simulink model "Single_Phase_Controlled_FWR_RLslx"  (R2025a)
settings: Solver=ode23tb  StartTime=0.0  StopTime=0.1  MaxStep=1e-4  RelTol=1e-3
libraries: spsThyristorLib x4, spsVoltageMeasurementLib x2, spsACVoltageSourceLib x1, spsCurrentMeasurementLib x1, spsDiodeLib x1, spsMeanLib x1, spsSeriesRLCBranchLib x1, sps_lib x1
settings Model: Creator=Jawad  LastModifiedBy=Jawad

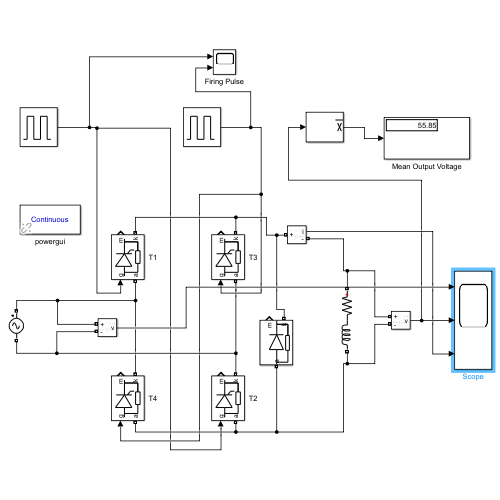
[thumbnail: Simulink's stored preview of the top-level diagram]
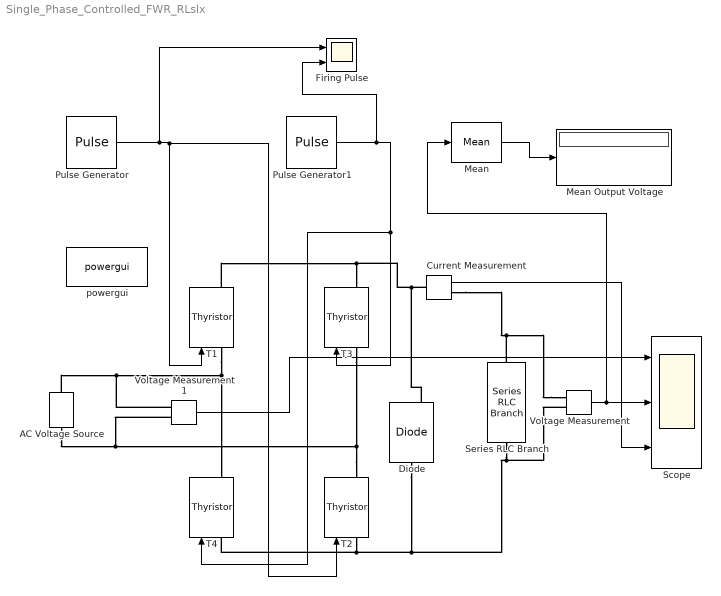
== system Single_Phase_Controlled_FWR_RLslx ==
  AC Voltage Source : spsACVoltageSourceLib/AC Voltage Source  Amplitude=100  Phase=0  Frequency=50  SampleTime=0  Measurements=None  BusType=swing  Pref=10e3  Qref=0  Qmin=-inf  Qmax=+inf
  Current Measurement : spsCurrentMeasurementLib/Current Measurement  PhasorSimulation=off  OutputType=Complex  PSBequivalent=0
  Diode : spsDiodeLib/Diode  Ron=0.001  Lon=0  Vf=0.8  IC=0  UseSnubber=0  Rs=500  Cs=250e-9  Measurements=on
  Firing Pulse : Scope  NumInputPorts=2
      settings: Title=FP_2  ActiveDisplayYMinimum=-0.62499999999999989  ActiveDisplayYMaximum=5.625
  Mean : spsMeanLib/Mean  Freq=60  Vinit=0  Ts=0
  Mean Output Voltage : Display
  Pulse Generator : DiscretePulseGenerator  PulseType=Time based  Amplitude=5  Period=0.02  PulseWidth=5  PhaseDelay=60*(0.02/360)
  Pulse Generator1 : DiscretePulseGenerator  PulseType=Time based  Amplitude=5  Period=0.02  PulseWidth=5  PhaseDelay=240*(0.02/360)
  Scope : Scope  NumInputPorts=3
      settings: ActiveDisplayString=3  Title=Io  ActiveDisplayYMinimum=-0.772150921983081  ActiveDisplayYMaximum=6.94935829784773
  Series RLC Branch : spsSeriesRLCBranchLib/Series RLC Branch  LConnTagsString=__new0  RConnTagsString=__new0  BranchType=RL  Resistance=10  Inductance=50e-3  SetiL0=off  InitialCurrent=0  Capacitance=1e-6  Setx0=off  InitialVoltage=0  Measurements=None
  T{1..4} (4 alike) : spsThyristorLib/Thyristor  Ron=0.001  Lon=0  Vf=0.8  IC=0  Rs=500  Cs=250e-9  Measurements=on
  Voltage Measurement : spsVoltageMeasurementLib/Voltage Measurement  PhasorSimulation=off  OutputType=Complex  PSBequivalent=0
  Voltage Measurement1 : spsVoltageMeasurementLib/Voltage Measurement  PhasorSimulation=off  OutputType=Complex  PSBequivalent=0
  powergui : sps_lib/powergui  Priority=1  SimulationMode=Continuous  SampleTime=50e-6  frequency=60  Iterations=50  frequencyindice=50  Pbase=100e6  ErrMax=1e-4  UnitsV=kV  UnitsW=MW  buscounter=0  FunctionMessages=off  echomessages=off  EnableUseOfTLC=off  CurrentSourceSwitches=off  DisableSnubberDevices=off  DisableRonSwitches=off  DisableVfSwitches=off  DisplayEquations=off  AutomaticDiscreteSolvers=off  SolverType=Tustin/Backward Euler (TBE)  Interpol=off  ExternalGateDelay=off  methode=off  Ts=100  x0status=blocks  SPID=on  SwTol=0  HookPort=off  NonlinearTolerance=1e-4  nMaxIteration=100  ContinueOnMaxIteration=off  RestoreLinks=warning  ResistiveCurrentMeasurement=off  Frange=[0:2:500]  Ylog=off  Xlog=on  ShowGrid=off  save=off  variable=ZData  structure=0  ZoomFFT=off  StartTime=0.0  cycles=1  DisplayStyle=1  fundamental=60  FreqAxis=off  MaxFrequency=1000  frequencyindicesteady=1  RmsSteady=1  display=off
  wires:
  Mean/1 -> Mean Output Voltage/1
  Pulse Generator1/1 -> Firing Pulse/2, T4/1, T3/1
  Voltage Measurement/1 -> Mean/1, Scope/2
  Voltage Measurement1/1 -> Scope/1
  Current Measurement/1 -> Scope/3
  Pulse Generator/1 -> Firing Pulse/1, T2/1, T1/1
  connections:
  T2/RConn1 -- T3/LConn1 -- Voltage Measurement1/LConn2 -- AC Voltage Source/LConn1
  Voltage Measurement/LConn2 -- Diode/LConn1 -- T2/LConn1 -- T4/LConn1 -- Series RLC Branch/RConn1
  AC Voltage Source/RConn1 -- T1/LConn1 -- T4/RConn1 -- Voltage Measurement1/LConn1
  Current Measurement/LConn1 -- T1/RConn1 -- T3/RConn1 -- Diode/RConn1
  Voltage Measurement/LConn1 -- Current Measurement/RConn1 -- Series RLC Branch/LConn1
